simulink model "Excersise3"  (R2023a)
settings: Solver=ode45  StartTime=0.0  StopTime=10.0  RelTol=1e-3
values from neighbouring files (symbols this model uses):
  A = [0 1 0 0 ... (first row only)    [invpendulum.m]
  B = [0; -(1/M*L); 0; 1/M]    [invpendulum.m]
  C = [1 0 0 0; 0 0 1 0;]    [invpendulum.m]
  D = [0; 0; 0; 0]    [invpendulum.m]
  F = -acker(A, B, poles_desired)    [invpendulum.m]
  K_fast = place(A.',C.',poles_fast).'    [invpendulum.m]
  x_0 = [0.1; 0; 0.1; 0]    [invpendulum.m]
settings Model: Creator=ioloizou  LastModifiedBy=ioloizou
settings DataIOCC: Refine=4

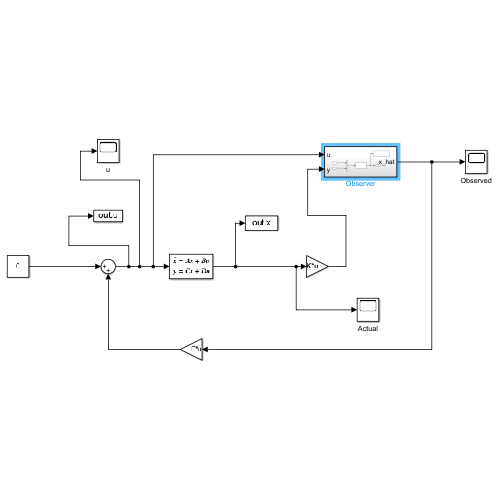
[thumbnail: Simulink's stored preview of the top-level diagram]
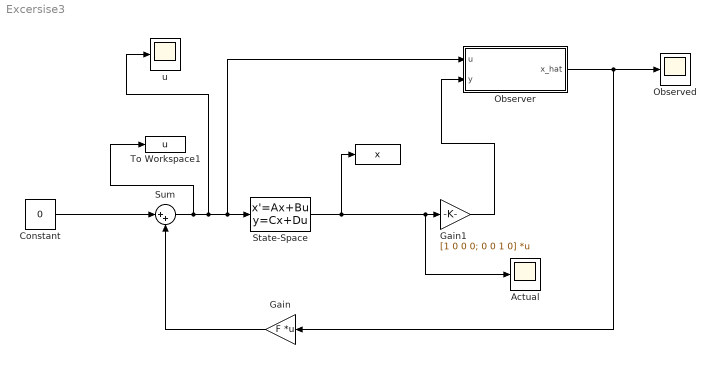
== system Excersise3 ==
  "  " : ToWorkspace  VariableName=x  SampleTime=-1
      settings: Save2DSignal=2-D array (concatenate along first dimension)
  Actual : Scope
  Constant : Constant  Value=0
  Gain : Gain  Gain=F  Multiplication=Matrix(K*u)
  Gain1 : Gain  Gain=[1 0 0 0; 0 0 1 0]  Multiplication=Matrix(K*u)
  Observed : Scope
  Observer : Subsystem
  State-Space : StateSpace  A=A  B=B  C=eye(4)  D=D  InitialCondition=x_0  ParameterTunability=Unconstrained
  Sum : Sum  Inputs=|++
  To Workspace1 : ToWorkspace  VariableName=u  SampleTime=-1
      settings: Save2DSignal=2-D array (concatenate along first dimension)
  u : Scope
  wires:
  Observer/1(x_hat) -> Gain/1, Observed/1
  Gain1/1 -> Observer/2(y)
  Gain/1 -> Sum/2
  State-Space/1 -> "  "/1, Actual/1, Gain1/1
  Sum/1 -> u/1, Observer/1(u), State-Space/1, To Workspace1/1
  Constant/1 -> Sum/1

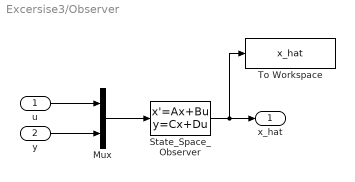
== system Excersise3/Observer ==
  u : Inport
  y : Inport  Port=2
  Mux : Mux  Inputs=2
  State_Space_Observer : StateSpace  A=A-K_fast*C  B=[B K_fast]  C=eye(4)  D=zeros(4,3)  InitialCondition=0
  To Workspace : ToWorkspace  VariableName=x_hat  SampleTime=-1
  x_hat : Outport
  wires:
  u/1 -> Mux/1
  y/1 -> Mux/2
  Mux/1 -> State_Space_Observer/1
  State_Space_Observer/1 -> To Workspace/1, x_hat/1
